simulink model "Problem2_BDA_DeClaroAndManimtim"  (R2023b)
settings: Solver=VariableStepAuto  StartTime=0.0  StopTime=20  RelTol=1e-3
values from neighbouring files (symbols this model uses):
  G1_den = [1 0 0]    [Problem2_DeClaroAndManimtim.m]
  G1_num = [1]    [Problem2_DeClaroAndManimtim.m]
  G2_den = [1 1]    [Problem2_DeClaroAndManimtim.m]
  G2_num = [1]    [Problem2_DeClaroAndManimtim.m]
  G3_den = [1 0]    [Problem2_DeClaroAndManimtim.m]
  G3_num = [1]    [Problem2_DeClaroAndManimtim.m]
  G4_den = [2 0]    [Problem2_DeClaroAndManimtim.m]
  G4_num = [1]    [Problem2_DeClaroAndManimtim.m]
  H1_den = [1 0]    [Problem2_DeClaroAndManimtim.m]
  H1_num = [1]    [Problem2_DeClaroAndManimtim.m]
  H2_den = [1 -1]    [Problem2_DeClaroAndManimtim.m]
  H2_num = [1]    [Problem2_DeClaroAndManimtim.m]
  H3_den = [1 -2]    [Problem2_DeClaroAndManimtim.m]
  H3_num = [1]    [Problem2_DeClaroAndManimtim.m]
  TF3_den = conv(G1G4TF2_den_H1_den_G1G4TF2_num_H1_num_sum, G1G4TF2_den)    [Problem2_DeClaroAndManimtim.m]
  TF3_num = conv(G1G4TF2_num_G1G4TF2_den, H1_den)    [Problem2_DeClaroAndManimtim.m]
settings Model: Creator=John Kenneth  LastModifiedBy=John Kenneth

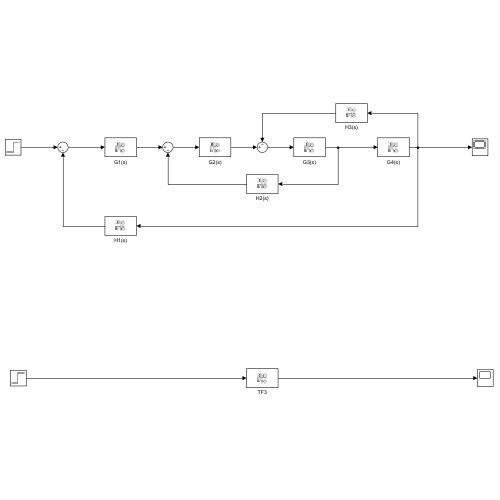
[thumbnail: Simulink's stored preview of the top-level diagram]
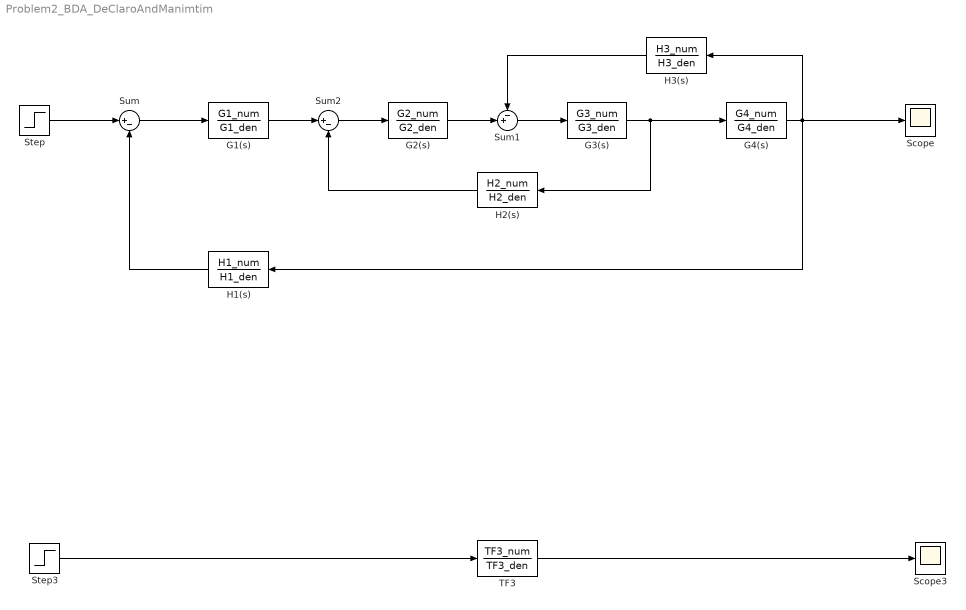
== system Problem2_BDA_DeClaroAndManimtim ==
  G1(s) : TransferFcn  Numerator=G1_num  Denominator=G1_den
  G2(s) : TransferFcn  Numerator=G2_num  Denominator=G2_den
  G3(s) : TransferFcn  Numerator=G3_num  Denominator=G3_den
  G4(s) : TransferFcn  Numerator=G4_num  Denominator=G4_den
  H1(s) : TransferFcn  Numerator=H1_num  Denominator=H1_den
  H2(s) : TransferFcn  Numerator=H2_num  Denominator=H2_den
  H3(s) : TransferFcn  Numerator=H3_num  Denominator=H3_den
  Scope : Scope
  Scope3 : Scope
  Step : Step  Time=0  SampleTime=0
  Step3 : Step  Time=0  SampleTime=0
  Sum : Sum  Inputs=|+-
  Sum1 : Sum  Inputs=-+|
  Sum2 : Sum  Inputs=|+-
  TF3 : TransferFcn  Numerator=TF3_num  Denominator=TF3_den
  wires:
  Step/1 -> Sum/1
  Sum/1 -> G1(s)/1
  G1(s)/1 -> Sum2/1
  Sum2/1 -> G2(s)/1
  G2(s)/1 -> Sum1/2
  Sum1/1 -> G3(s)/1
  H3(s)/1 -> Sum1/1
  G3(s)/1 -> H2(s)/1, G4(s)/1
  H2(s)/1 -> Sum2/2
  H1(s)/1 -> Sum/2
  G4(s)/1 -> H1(s)/1, Scope/1, H3(s)/1
  Step3/1 -> TF3/1
  TF3/1 -> Scope3/1
